simulink model "Beautiful_powertrain"  (R2024a)
settings: Solver=ode3  StartTime=0.0  StopTime=40  FixedStep=0.001  RelTol=1e-3
model workspace (MAT data in the model file):
  C_Aero_drag = 0.28
  C_rolling_resistance = 0.01
  C_rolling_resitance = 0.01
  C_viscous_damping = 0.02
  Damping_coef = 50
  Gear_ratio = 10
  J_vehicle = 2.56328
  Motor_no_load_speed = 16000
  Motor_rated_load = 150000
  Motor_rated_speed = 9000
  Motor_rotor_damping = 0.02
  Motor_rotor_inertia = 0.05
  Motor_voltage = 450
  Slope = 0
  Vehicle_Wheel_Radius = 0.358
  Vehicle_frontal_area = 2.56
  Vehicle_mass = 2000
values from neighbouring files (symbols this model uses):
  s = sprintf('    [N_diangostic_2.m]
undefined symbols (not defined in the file or in its folder): battery_builder_rtmsupport, gcbh
libraries: Batteries_lib x36, fl_lib x31, nesl_utility x24, ee_lib x3, autolibshared x2, rllib x2, sdl_lib x1
(part 2 of 6)

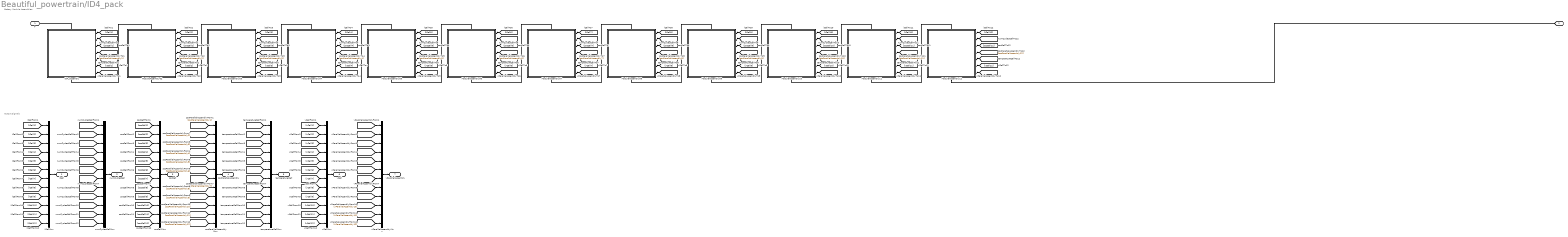
== system Beautiful_powertrain/ID4_pack ==
  note: Output Signals
  note: Battery Module Assemblies
  ID4_Assembly : Subsystem  LoadFcn=battery_builder_rtmsupport('loadfcn',gcbh);
      settings: CopyFcn=battery_builder_rtmsupport('copyfcn',gcbh);  PreCopyFcn=battery_builder_rtmsupport('precopyfcn',gcbh);  PreDeleteFcn=battery_builder_rtmsupport('predeletefcn',gcbh);  PortSchema="{\"entries\":[{\"content\":{\"sides\":[{\"content\":{\"connectorIds\":[\"LConn1\"]},\"type\":\"ConnectorPlacement.EquallySpacedRectSide\",\"uuid\":\"ff832d46-24c2-48f3-9ca2-acbc79ffea0e\"},{\"content\":{\"connectorIds\":[\"RConn1\"],\"side\":\"RIGHT\"},\"type\":\"ConnectorPlacement.EquallySpacedRectSide\",\"uuid\":\"f1f3b13c-36d9-4e7c-bb66-ad6aba201785\"},{\"content\":{\"side\":\"TOP\"},\"type\":\"ConnectorPlacement.EquallySpacedRectSide\",\"uuid\":\"497ed55c-0d21-4aaa-b04e-04d199c99403\"},{\"content\":{\"connectorIds\":[\"Out1\",\"Out2\",\"Out3\",\"Out4\",\"Out5\",\"Out6\",\"Out7\"],\"side\":\"BOTTOM\"},\"type\":\"ConnectorPlacement.EquallySpacedRectSide\",\"uuid\":\"076cd1de-5daa-42e2-9426-d52e4d178271\"}]},\"type\":\"ConnectorPlacement.EquallySpacedConnector\",\"uuid\":\"b44e404e-c709-4efd-83da-0fbfd4cccfd0\"}],\"packageUris\":[\"http://schema.mathworks.com/mf0/Connector/R2020b\"],\"version\":\"1.0\"}"
      mask Display: image('$imagefile')
  ModuleAssembly02 : Subsystem  LoadFcn=battery_builder_rtmsupport('loadfcn',gcbh);
      settings: CopyFcn=battery_builder_rtmsupport('copyfcn',gcbh);  PreCopyFcn=battery_builder_rtmsupport('precopyfcn',gcbh);  PreDeleteFcn=battery_builder_rtmsupport('predeletefcn',gcbh);  PortSchema="{\"entries\":[{\"content\":{\"sides\":[{\"content\":{\"connectorIds\":[\"LConn1\"]},\"type\":\"ConnectorPlacement.EquallySpacedRectSide\",\"uuid\":\"ff832d46-24c2-48f3-9ca2-acbc79ffea0e\"},{\"content\":{\"connectorIds\":[\"RConn1\"],\"side\":\"RIGHT\"},\"type\":\"ConnectorPlacement.EquallySpacedRectSide\",\"uuid\":\"f1f3b13c-36d9-4e7c-bb66-ad6aba201785\"},{\"content\":{\"side\":\"TOP\"},\"type\":\"ConnectorPlacement.EquallySpacedRectSide\",\"uuid\":\"497ed55c-0d21-4aaa-b04e-04d199c99403\"},{\"content\":{\"connectorIds\":[\"Out1\",\"Out2\",\"Out3\",\"Out4\",\"Out5\",\"Out6\",\"Out7\"],\"side\":\"BOTTOM\"},\"type\":\"ConnectorPlacement.EquallySpacedRectSide\",\"uuid\":\"076cd1de-5daa-42e2-9426-d52e4d178271\"}]},\"type\":\"ConnectorPlacement.EquallySpacedConnector\",\"uuid\":\"b44e404e-c709-4efd-83da-0fbfd4cccfd0\"}],\"packageUris\":[\"http://schema.mathworks.com/mf0/Connector/R2020b\"],\"version\":\"1.0\"}"
      mask Display: image('$imagefile')
  ModuleAssembly03 : Subsystem  LoadFcn=battery_builder_rtmsupport('loadfcn',gcbh);
      settings: CopyFcn=battery_builder_rtmsupport('copyfcn',gcbh);  PreCopyFcn=battery_builder_rtmsupport('precopyfcn',gcbh);  PreDeleteFcn=battery_builder_rtmsupport('predeletefcn',gcbh);  PortSchema="{\"entries\":[{\"content\":{\"sides\":[{\"content\":{\"connectorIds\":[\"LConn1\"]},\"type\":\"ConnectorPlacement.EquallySpacedRectSide\",\"uuid\":\"ff832d46-24c2-48f3-9ca2-acbc79ffea0e\"},{\"content\":{\"connectorIds\":[\"RConn1\"],\"side\":\"RIGHT\"},\"type\":\"ConnectorPlacement.EquallySpacedRectSide\",\"uuid\":\"f1f3b13c-36d9-4e7c-bb66-ad6aba201785\"},{\"content\":{\"side\":\"TOP\"},\"type\":\"ConnectorPlacement.EquallySpacedRectSide\",\"uuid\":\"497ed55c-0d21-4aaa-b04e-04d199c99403\"},{\"content\":{\"connectorIds\":[\"Out1\",\"Out2\",\"Out3\",\"Out4\",\"Out5\",\"Out6\",\"Out7\"],\"side\":\"BOTTOM\"},\"type\":\"ConnectorPlacement.EquallySpacedRectSide\",\"uuid\":\"076cd1de-5daa-42e2-9426-d52e4d178271\"}]},\"type\":\"ConnectorPlacement.EquallySpacedConnector\",\"uuid\":\"b44e404e-c709-4efd-83da-0fbfd4cccfd0\"}],\"packageUris\":[\"http://schema.mathworks.com/mf0/Connector/R2020b\"],\"version\":\"1.0\"}"
      mask Display: image('$imagefile')
  ModuleAssembly04 : Subsystem  LoadFcn=battery_builder_rtmsupport('loadfcn',gcbh);
      settings: CopyFcn=battery_builder_rtmsupport('copyfcn',gcbh);  PreCopyFcn=battery_builder_rtmsupport('precopyfcn',gcbh);  PreDeleteFcn=battery_builder_rtmsupport('predeletefcn',gcbh);  PortSchema="{\"entries\":[{\"content\":{\"sides\":[{\"content\":{\"connectorIds\":[\"LConn1\"]},\"type\":\"ConnectorPlacement.EquallySpacedRectSide\",\"uuid\":\"ff832d46-24c2-48f3-9ca2-acbc79ffea0e\"},{\"content\":{\"connectorIds\":[\"RConn1\"],\"side\":\"RIGHT\"},\"type\":\"ConnectorPlacement.EquallySpacedRectSide\",\"uuid\":\"f1f3b13c-36d9-4e7c-bb66-ad6aba201785\"},{\"content\":{\"side\":\"TOP\"},\"type\":\"ConnectorPlacement.EquallySpacedRectSide\",\"uuid\":\"497ed55c-0d21-4aaa-b04e-04d199c99403\"},{\"content\":{\"connectorIds\":[\"Out1\",\"Out2\",\"Out3\",\"Out4\",\"Out5\",\"Out6\",\"Out7\"],\"side\":\"BOTTOM\"},\"type\":\"ConnectorPlacement.EquallySpacedRectSide\",\"uuid\":\"076cd1de-5daa-42e2-9426-d52e4d178271\"}]},\"type\":\"ConnectorPlacement.EquallySpacedConnector\",\"uuid\":\"b44e404e-c709-4efd-83da-0fbfd4cccfd0\"}],\"packageUris\":[\"http://schema.mathworks.com/mf0/Connector/R2020b\"],\"version\":\"1.0\"}"
      mask Display: image('$imagefile')
  ModuleAssembly05 : Subsystem  LoadFcn=battery_builder_rtmsupport('loadfcn',gcbh);
      settings: CopyFcn=battery_builder_rtmsupport('copyfcn',gcbh);  PreCopyFcn=battery_builder_rtmsupport('precopyfcn',gcbh);  PreDeleteFcn=battery_builder_rtmsupport('predeletefcn',gcbh);  PortSchema="{\"entries\":[{\"content\":{\"sides\":[{\"content\":{\"connectorIds\":[\"LConn1\"]},\"type\":\"ConnectorPlacement.EquallySpacedRectSide\",\"uuid\":\"ff832d46-24c2-48f3-9ca2-acbc79ffea0e\"},{\"content\":{\"connectorIds\":[\"RConn1\"],\"side\":\"RIGHT\"},\"type\":\"ConnectorPlacement.EquallySpacedRectSide\",\"uuid\":\"f1f3b13c-36d9-4e7c-bb66-ad6aba201785\"},{\"content\":{\"side\":\"TOP\"},\"type\":\"ConnectorPlacement.EquallySpacedRectSide\",\"uuid\":\"497ed55c-0d21-4aaa-b04e-04d199c99403\"},{\"content\":{\"connectorIds\":[\"Out1\",\"Out2\",\"Out3\",\"Out4\",\"Out5\",\"Out6\",\"Out7\"],\"side\":\"BOTTOM\"},\"type\":\"ConnectorPlacement.EquallySpacedRectSide\",\"uuid\":\"076cd1de-5daa-42e2-9426-d52e4d178271\"}]},\"type\":\"ConnectorPlacement.EquallySpacedConnector\",\"uuid\":\"b44e404e-c709-4efd-83da-0fbfd4cccfd0\"}],\"packageUris\":[\"http://schema.mathworks.com/mf0/Connector/R2020b\"],\"version\":\"1.0\"}"
      mask Display: image('$imagefile')
  ModuleAssembly06 : Subsystem  LoadFcn=battery_builder_rtmsupport('loadfcn',gcbh);
      settings: CopyFcn=battery_builder_rtmsupport('copyfcn',gcbh);  PreCopyFcn=battery_builder_rtmsupport('precopyfcn',gcbh);  PreDeleteFcn=battery_builder_rtmsupport('predeletefcn',gcbh);  PortSchema="{\"entries\":[{\"content\":{\"sides\":[{\"content\":{\"connectorIds\":[\"LConn1\"]},\"type\":\"ConnectorPlacement.EquallySpacedRectSide\",\"uuid\":\"ff832d46-24c2-48f3-9ca2-acbc79ffea0e\"},{\"content\":{\"connectorIds\":[\"RConn1\"],\"side\":\"RIGHT\"},\"type\":\"ConnectorPlacement.EquallySpacedRectSide\",\"uuid\":\"f1f3b13c-36d9-4e7c-bb66-ad6aba201785\"},{\"content\":{\"side\":\"TOP\"},\"type\":\"ConnectorPlacement.EquallySpacedRectSide\",\"uuid\":\"497ed55c-0d21-4aaa-b04e-04d199c99403\"},{\"content\":{\"connectorIds\":[\"Out1\",\"Out2\",\"Out3\",\"Out4\",\"Out5\",\"Out6\",\"Out7\"],\"side\":\"BOTTOM\"},\"type\":\"ConnectorPlacement.EquallySpacedRectSide\",\"uuid\":\"076cd1de-5daa-42e2-9426-d52e4d178271\"}]},\"type\":\"ConnectorPlacement.EquallySpacedConnector\",\"uuid\":\"b44e404e-c709-4efd-83da-0fbfd4cccfd0\"}],\"packageUris\":[\"http://schema.mathworks.com/mf0/Connector/R2020b\"],\"version\":\"1.0\"}"
      mask Display: image('$imagefile')
  ModuleAssembly07 : Subsystem  LoadFcn=battery_builder_rtmsupport('loadfcn',gcbh);
      settings: CopyFcn=battery_builder_rtmsupport('copyfcn',gcbh);  PreCopyFcn=battery_builder_rtmsupport('precopyfcn',gcbh);  PreDeleteFcn=battery_builder_rtmsupport('predeletefcn',gcbh);  PortSchema="{\"entries\":[{\"content\":{\"sides\":[{\"content\":{\"connectorIds\":[\"LConn1\"]},\"type\":\"ConnectorPlacement.EquallySpacedRectSide\",\"uuid\":\"ff832d46-24c2-48f3-9ca2-acbc79ffea0e\"},{\"content\":{\"connectorIds\":[\"RConn1\"],\"side\":\"RIGHT\"},\"type\":\"ConnectorPlacement.EquallySpacedRectSide\",\"uuid\":\"f1f3b13c-36d9-4e7c-bb66-ad6aba201785\"},{\"content\":{\"side\":\"TOP\"},\"type\":\"ConnectorPlacement.EquallySpacedRectSide\",\"uuid\":\"497ed55c-0d21-4aaa-b04e-04d199c99403\"},{\"content\":{\"connectorIds\":[\"Out1\",\"Out2\",\"Out3\",\"Out4\",\"Out5\",\"Out6\",\"Out7\"],\"side\":\"BOTTOM\"},\"type\":\"ConnectorPlacement.EquallySpacedRectSide\",\"uuid\":\"076cd1de-5daa-42e2-9426-d52e4d178271\"}]},\"type\":\"ConnectorPlacement.EquallySpacedConnector\",\"uuid\":\"b44e404e-c709-4efd-83da-0fbfd4cccfd0\"}],\"packageUris\":[\"http://schema.mathworks.com/mf0/Connector/R2020b\"],\"version\":\"1.0\"}"
      mask Display: image('$imagefile')
  ModuleAssembly08 : Subsystem  LoadFcn=battery_builder_rtmsupport('loadfcn',gcbh);
      settings: CopyFcn=battery_builder_rtmsupport('copyfcn',gcbh);  PreCopyFcn=battery_builder_rtmsupport('precopyfcn',gcbh);  PreDeleteFcn=battery_builder_rtmsupport('predeletefcn',gcbh);  PortSchema="{\"entries\":[{\"content\":{\"sides\":[{\"content\":{\"connectorIds\":[\"LConn1\"]},\"type\":\"ConnectorPlacement.EquallySpacedRectSide\",\"uuid\":\"ff832d46-24c2-48f3-9ca2-acbc79ffea0e\"},{\"content\":{\"connectorIds\":[\"RConn1\"],\"side\":\"RIGHT\"},\"type\":\"ConnectorPlacement.EquallySpacedRectSide\",\"uuid\":\"f1f3b13c-36d9-4e7c-bb66-ad6aba201785\"},{\"content\":{\"side\":\"TOP\"},\"type\":\"ConnectorPlacement.EquallySpacedRectSide\",\"uuid\":\"497ed55c-0d21-4aaa-b04e-04d199c99403\"},{\"content\":{\"connectorIds\":[\"Out1\",\"Out2\",\"Out3\",\"Out4\",\"Out5\",\"Out6\",\"Out7\"],\"side\":\"BOTTOM\"},\"type\":\"ConnectorPlacement.EquallySpacedRectSide\",\"uuid\":\"076cd1de-5daa-42e2-9426-d52e4d178271\"}]},\"type\":\"ConnectorPlacement.EquallySpacedConnector\",\"uuid\":\"b44e404e-c709-4efd-83da-0fbfd4cccfd0\"}],\"packageUris\":[\"http://schema.mathworks.com/mf0/Connector/R2020b\"],\"version\":\"1.0\"}"
      mask Display: image('$imagefile')
  ModuleAssembly09 : Subsystem  LoadFcn=battery_builder_rtmsupport('loadfcn',gcbh);
      settings: CopyFcn=battery_builder_rtmsupport('copyfcn',gcbh);  PreCopyFcn=battery_builder_rtmsupport('precopyfcn',gcbh);  PreDeleteFcn=battery_builder_rtmsupport('predeletefcn',gcbh);  PortSchema="{\"entries\":[{\"content\":{\"sides\":[{\"content\":{\"connectorIds\":[\"LConn1\"]},\"type\":\"ConnectorPlacement.EquallySpacedRectSide\",\"uuid\":\"ff832d46-24c2-48f3-9ca2-acbc79ffea0e\"},{\"content\":{\"connectorIds\":[\"RConn1\"],\"side\":\"RIGHT\"},\"type\":\"ConnectorPlacement.EquallySpacedRectSide\",\"uuid\":\"f1f3b13c-36d9-4e7c-bb66-ad6aba201785\"},{\"content\":{\"side\":\"TOP\"},\"type\":\"ConnectorPlacement.EquallySpacedRectSide\",\"uuid\":\"497ed55c-0d21-4aaa-b04e-04d199c99403\"},{\"content\":{\"connectorIds\":[\"Out1\",\"Out2\",\"Out3\",\"Out4\",\"Out5\",\"Out6\",\"Out7\"],\"side\":\"BOTTOM\"},\"type\":\"ConnectorPlacement.EquallySpacedRectSide\",\"uuid\":\"076cd1de-5daa-42e2-9426-d52e4d178271\"}]},\"type\":\"ConnectorPlacement.EquallySpacedConnector\",\"uuid\":\"b44e404e-c709-4efd-83da-0fbfd4cccfd0\"}],\"packageUris\":[\"http://schema.mathworks.com/mf0/Connector/R2020b\"],\"version\":\"1.0\"}"
      mask Display: image('$imagefile')
  ModuleAssembly10 : Subsystem  LoadFcn=battery_builder_rtmsupport('loadfcn',gcbh);
      settings: CopyFcn=battery_builder_rtmsupport('copyfcn',gcbh);  PreCopyFcn=battery_builder_rtmsupport('precopyfcn',gcbh);  PreDeleteFcn=battery_builder_rtmsupport('predeletefcn',gcbh);  PortSchema="{\"entries\":[{\"content\":{\"sides\":[{\"content\":{\"connectorIds\":[\"LConn1\"]},\"type\":\"ConnectorPlacement.EquallySpacedRectSide\",\"uuid\":\"ff832d46-24c2-48f3-9ca2-acbc79ffea0e\"},{\"content\":{\"connectorIds\":[\"RConn1\"],\"side\":\"RIGHT\"},\"type\":\"ConnectorPlacement.EquallySpacedRectSide\",\"uuid\":\"f1f3b13c-36d9-4e7c-bb66-ad6aba201785\"},{\"content\":{\"side\":\"TOP\"},\"type\":\"ConnectorPlacement.EquallySpacedRectSide\",\"uuid\":\"497ed55c-0d21-4aaa-b04e-04d199c99403\"},{\"content\":{\"connectorIds\":[\"Out1\",\"Out2\",\"Out3\",\"Out4\",\"Out5\",\"Out6\",\"Out7\"],\"side\":\"BOTTOM\"},\"type\":\"ConnectorPlacement.EquallySpacedRectSide\",\"uuid\":\"076cd1de-5daa-42e2-9426-d52e4d178271\"}]},\"type\":\"ConnectorPlacement.EquallySpacedConnector\",\"uuid\":\"b44e404e-c709-4efd-83da-0fbfd4cccfd0\"}],\"packageUris\":[\"http://schema.mathworks.com/mf0/Connector/R2020b\"],\"version\":\"1.0\"}"
      mask Display: image('$imagefile')
  ModuleAssembly11 : Subsystem  LoadFcn=battery_builder_rtmsupport('loadfcn',gcbh);
      settings: CopyFcn=battery_builder_rtmsupport('copyfcn',gcbh);  PreCopyFcn=battery_builder_rtmsupport('precopyfcn',gcbh);  PreDeleteFcn=battery_builder_rtmsupport('predeletefcn',gcbh);  PortSchema="{\"entries\":[{\"content\":{\"sides\":[{\"content\":{\"connectorIds\":[\"LConn1\"]},\"type\":\"ConnectorPlacement.EquallySpacedRectSide\",\"uuid\":\"ff832d46-24c2-48f3-9ca2-acbc79ffea0e\"},{\"content\":{\"connectorIds\":[\"RConn1\"],\"side\":\"RIGHT\"},\"type\":\"ConnectorPlacement.EquallySpacedRectSide\",\"uuid\":\"f1f3b13c-36d9-4e7c-bb66-ad6aba201785\"},{\"content\":{\"side\":\"TOP\"},\"type\":\"ConnectorPlacement.EquallySpacedRectSide\",\"uuid\":\"497ed55c-0d21-4aaa-b04e-04d199c99403\"},{\"content\":{\"connectorIds\":[\"Out1\",\"Out2\",\"Out3\",\"Out4\",\"Out5\",\"Out6\",\"Out7\"],\"side\":\"BOTTOM\"},\"type\":\"ConnectorPlacement.EquallySpacedRectSide\",\"uuid\":\"076cd1de-5daa-42e2-9426-d52e4d178271\"}]},\"type\":\"ConnectorPlacement.EquallySpacedConnector\",\"uuid\":\"b44e404e-c709-4efd-83da-0fbfd4cccfd0\"}],\"packageUris\":[\"http://schema.mathworks.com/mf0/Connector/R2020b\"],\"version\":\"1.0\"}"
      mask Display: image('$imagefile')
  ModuleAssembly12 : Subsystem  LoadFcn=battery_builder_rtmsupport('loadfcn',gcbh);
      settings: CopyFcn=battery_builder_rtmsupport('copyfcn',gcbh);  PreCopyFcn=battery_builder_rtmsupport('precopyfcn',gcbh);  PreDeleteFcn=battery_builder_rtmsupport('predeletefcn',gcbh);  PortSchema="{\"entries\":[{\"content\":{\"sides\":[{\"content\":{\"connectorIds\":[\"LConn1\"]},\"type\":\"ConnectorPlacement.EquallySpacedRectSide\",\"uuid\":\"ff832d46-24c2-48f3-9ca2-acbc79ffea0e\"},{\"content\":{\"connectorIds\":[\"RConn1\"],\"side\":\"RIGHT\"},\"type\":\"ConnectorPlacement.EquallySpacedRectSide\",\"uuid\":\"f1f3b13c-36d9-4e7c-bb66-ad6aba201785\"},{\"content\":{\"side\":\"TOP\"},\"type\":\"ConnectorPlacement.EquallySpacedRectSide\",\"uuid\":\"497ed55c-0d21-4aaa-b04e-04d199c99403\"},{\"content\":{\"connectorIds\":[\"Out1\",\"Out2\",\"Out3\",\"Out4\",\"Out5\",\"Out6\",\"Out7\"],\"side\":\"BOTTOM\"},\"type\":\"ConnectorPlacement.EquallySpacedRectSide\",\"uuid\":\"076cd1de-5daa-42e2-9426-d52e4d178271\"}]},\"type\":\"ConnectorPlacement.EquallySpacedConnector\",\"uuid\":\"b44e404e-c709-4efd-83da-0fbfd4cccfd0\"}],\"packageUris\":[\"http://schema.mathworks.com/mf0/Connector/R2020b\"],\"version\":\"1.0\"}"
      mask Display: image('$imagefile')
  iCellMux : Mux  Inputs=12
  numCyclesCellMux : Mux  Inputs=12
  socCellMux : Mux  Inputs=12
  socParallelAssemblyMux : Mux  Inputs=12
  temperatureCellMux : Mux  Inputs=12
  vCellMux : Mux  Inputs=12
  vParallelAssemblyMux : Mux  Inputs=12
  + : PMIOPort  Side=Left
  - : PMIOPort  Port=2  Side=Right
  iCell : Outport
  numCyclesCell : Outport  Port=2
  socCell : Outport  Port=3
  socParallelAssembly : Outport  Port=4
  temperatureCell : Outport  Port=5
  vCell : Outport  Port=6
  vParallelAssembly : Outport  Port=7
  wires:
  [vParallelAssembly12] -> vParallelAssemblyMux/12
  ModuleAssembly12/7(vParallelAssembly) -> [vParallelAssembly12]
  [vCell12] -> vCellMux/12
  ModuleAssembly12/6(vCell) -> [vCell12]
  [temperatureCell12] -> temperatureCellMux/12
  ModuleAssembly12/5(temperatureCell) -> [temperatureCell12]
  [socParallelAssembly12] -> socParallelAssemblyMux/12
  ModuleAssembly12/4(socParallelAssembly) -> [socParallelAssembly12]
  [socCell12] -> socCellMux/12
  ModuleAssembly12/3(socCell) -> [socCell12]
  [numCyclesCell12] -> numCyclesCellMux/12
  ModuleAssembly12/2(numCyclesCell) -> [numCyclesCell12]
  [iCell12] -> iCellMux/12
  ModuleAssembly12/1(iCell) -> [iCell12]
  [vParallelAssembly11] -> vParallelAssemblyMux/11
  ModuleAssembly11/7(vParallelAssembly) -> [vParallelAssembly11]
  [vCell11] -> vCellMux/11
  ModuleAssembly11/6(vCell) -> [vCell11]
  [temperatureCell11] -> temperatureCellMux/11
  ModuleAssembly11/5(temperatureCell) -> [temperatureCell11]
  [socParallelAssembly11] -> socParallelAssemblyMux/11
  ModuleAssembly11/4(socParallelAssembly) -> [socParallelAssembly11]
  [socCell11] -> socCellMux/11
  ModuleAssembly11/3(socCell) -> [socCell11]
  [numCyclesCell11] -> numCyclesCellMux/11
  ModuleAssembly11/2(numCyclesCell) -> [numCyclesCell11]
  [iCell11] -> iCellMux/11
  ModuleAssembly11/1(iCell) -> [iCell11]
  [vParallelAssembly10] -> vParallelAssemblyMux/10
  ModuleAssembly10/7(vParallelAssembly) -> [vParallelAssembly10]
  [vCell10] -> vCellMux/10
  ModuleAssembly10/6(vCell) -> [vCell10]
  [temperatureCell10] -> temperatureCellMux/10
  ModuleAssembly10/5(temperatureCell) -> [temperatureCell10]
  [socParallelAssembly10] -> socParallelAssemblyMux/10
  ModuleAssembly10/4(socParallelAssembly) -> [socParallelAssembly10]
  [socCell10] -> socCellMux/10
  ModuleAssembly10/3(socCell) -> [socCell10]
  [numCyclesCell10] -> numCyclesCellMux/10
  ModuleAssembly10/2(numCyclesCell) -> [numCyclesCell10]
  [iCell10] -> iCellMux/10
  ModuleAssembly10/1(iCell) -> [iCell10]
  [vParallelAssembly9] -> vParallelAssemblyMux/9
  ModuleAssembly09/7(vParallelAssembly) -> [vParallelAssembly9]
  [vCell9] -> vCellMux/9
  ModuleAssembly09/6(vCell) -> [vCell9]
  [temperatureCell9] -> temperatureCellMux/9
  ModuleAssembly09/5(temperatureCell) -> [temperatureCell9]
  [socParallelAssembly9] -> socParallelAssemblyMux/9
  ModuleAssembly09/4(socParallelAssembly) -> [socParallelAssembly9]
  [socCell9] -> socCellMux/9
  ModuleAssembly09/3(socCell) -> [socCell9]
  [numCyclesCell9] -> numCyclesCellMux/9
  ModuleAssembly09/2(numCyclesCell) -> [numCyclesCell9]
  [iCell9] -> iCellMux/9
  ModuleAssembly09/1(iCell) -> [iCell9]
  [vParallelAssembly8] -> vParallelAssemblyMux/8
  ModuleAssembly08/7(vParallelAssembly) -> [vParallelAssembly8]
  [vCell8] -> vCellMux/8
  ModuleAssembly08/6(vCell) -> [vCell8]
  [temperatureCell8] -> temperatureCellMux/8
  ModuleAssembly08/5(temperatureCell) -> [temperatureCell8]
  [socParallelAssembly8] -> socParallelAssemblyMux/8
  ModuleAssembly08/4(socParallelAssembly) -> [socParallelAssembly8]
  [socCell8] -> socCellMux/8
  ModuleAssembly08/3(socCell) -> [socCell8]
  [numCyclesCell8] -> numCyclesCellMux/8
  ModuleAssembly08/2(numCyclesCell) -> [numCyclesCell8]
  [iCell8] -> iCellMux/8
  ModuleAssembly08/1(iCell) -> [iCell8]
  [vParallelAssembly7] -> vParallelAssemblyMux/7
  ModuleAssembly07/7(vParallelAssembly) -> [vParallelAssembly7]
  [vCell7] -> vCellMux/7
  ModuleAssembly07/6(vCell) -> [vCell7]
  [temperatureCell7] -> temperatureCellMux/7
  ModuleAssembly07/5(temperatureCell) -> [temperatureCell7]
  [socParallelAssembly7] -> socParallelAssemblyMux/7
  ModuleAssembly07/4(socParallelAssembly) -> [socParallelAssembly7]
  [socCell7] -> socCellMux/7
  ModuleAssembly07/3(socCell) -> [socCell7]
  [numCyclesCell7] -> numCyclesCellMux/7
  ModuleAssembly07/2(numCyclesCell) -> [numCyclesCell7]
  [iCell7] -> iCellMux/7
  ModuleAssembly07/1(iCell) -> [iCell7]
  [vParallelAssembly6] -> vParallelAssemblyMux/6
  ModuleAssembly06/7(vParallelAssembly) -> [vParallelAssembly6]
  [vCell6] -> vCellMux/6
  ModuleAssembly06/6(vCell) -> [vCell6]
  [temperatureCell6] -> temperatureCellMux/6
  ModuleAssembly06/5(temperatureCell) -> [temperatureCell6]
  [socParallelAssembly6] -> socParallelAssemblyMux/6
  ModuleAssembly06/4(socParallelAssembly) -> [socParallelAssembly6]
  [socCell6] -> socCellMux/6
  ModuleAssembly06/3(socCell) -> [socCell6]
  [numCyclesCell6] -> numCyclesCellMux/6
  ModuleAssembly06/2(numCyclesCell) -> [numCyclesCell6]
  [iCell6] -> iCellMux/6
  ModuleAssembly06/1(iCell) -> [iCell6]
  [vParallelAssembly5] -> vParallelAssemblyMux/5
  ModuleAssembly05/7(vParallelAssembly) -> [vParallelAssembly5]
  [vCell5] -> vCellMux/5
  ModuleAssembly05/6(vCell) -> [vCell5]
  [temperatureCell5] -> temperatureCellMux/5
  ModuleAssembly05/5(temperatureCell) -> [temperatureCell5]
  [socParallelAssembly5] -> socParallelAssemblyMux/5
  ModuleAssembly05/4(socParallelAssembly) -> [socParallelAssembly5]
  [socCell5] -> socCellMux/5
  ModuleAssembly05/3(socCell) -> [socCell5]
  [numCyclesCell5] -> numCyclesCellMux/5
  ModuleAssembly05/2(numCyclesCell) -> [numCyclesCell5]
  [iCell5] -> iCellMux/5
  ModuleAssembly05/1(iCell) -> [iCell5]
  [vParallelAssembly4] -> vParallelAssemblyMux/4
  ModuleAssembly04/7(vParallelAssembly) -> [vParallelAssembly4]
  [vCell4] -> vCellMux/4
  ModuleAssembly04/6(vCell) -> [vCell4]
  [temperatureCell4] -> temperatureCellMux/4
  ModuleAssembly04/5(temperatureCell) -> [temperatureCell4]
  [socParallelAssembly4] -> socParallelAssemblyMux/4
  ModuleAssembly04/4(socParallelAssembly) -> [socParallelAssembly4]
  [socCell4] -> socCellMux/4
  ModuleAssembly04/3(socCell) -> [socCell4]
  [numCyclesCell4] -> numCyclesCellMux/4
  ModuleAssembly04/2(numCyclesCell) -> [numCyclesCell4]
  [iCell4] -> iCellMux/4
  ModuleAssembly04/1(iCell) -> [iCell4]
  [vParallelAssembly3] -> vParallelAssemblyMux/3
  ModuleAssembly03/7(vParallelAssembly) -> [vParallelAssembly3]
  [vCell3] -> vCellMux/3
  ModuleAssembly03/6(vCell) -> [vCell3]
  [temperatureCell3] -> temperatureCellMux/3
  ModuleAssembly03/5(temperatureCell) -> [temperatureCell3]
  [socParallelAssembly3] -> socParallelAssemblyMux/3
  ModuleAssembly03/4(socParallelAssembly) -> [socParallelAssembly3]
  [socCell3] -> socCellMux/3
  ModuleAssembly03/3(socCell) -> [socCell3]
  [numCyclesCell3] -> numCyclesCellMux/3
  ModuleAssembly03/2(numCyclesCell) -> [numCyclesCell3]
  [iCell3] -> iCellMux/3
  ModuleAssembly03/1(iCell) -> [iCell3]
  [vParallelAssembly2] -> vParallelAssemblyMux/2
  ModuleAssembly02/7(vParallelAssembly) -> [vParallelAssembly2]
  [vCell2] -> vCellMux/2
  ModuleAssembly02/6(vCell) -> [vCell2]
  [temperatureCell2] -> temperatureCellMux/2
  ModuleAssembly02/5(temperatureCell) -> [temperatureCell2]
  [socParallelAssembly2] -> socParallelAssemblyMux/2
  ModuleAssembly02/4(socParallelAssembly) -> [socParallelAssembly2]
  [socCell2] -> socCellMux/2
  ModuleAssembly02/3(socCell) -> [socCell2]
  [numCyclesCell2] -> numCyclesCellMux/2
  ModuleAssembly02/2(numCyclesCell) -> [numCyclesCell2]
  [iCell2] -> iCellMux/2
  ModuleAssembly02/1(iCell) -> [iCell2]
  [vParallelAssembly1] -> vParallelAssemblyMux/1
  vParallelAssemblyMux/1 -> vParallelAssembly/1
  ID4_Assembly/7(vParallelAssembly) -> [vParallelAssembly1]
  [vCell1] -> vCellMux/1
  vCellMux/1 -> vCell/1
  ID4_Assembly/6(vCell) -> [vCell1]
  [temperatureCell1] -> temperatureCellMux/1
  temperatureCellMux/1 -> temperatureCell/1
  ID4_Assembly/5(temperatureCell) -> [temperatureCell1]
  [socParallelAssembly1] -> socParallelAssemblyMux/1
  socParallelAssemblyMux/1 -> socParallelAssembly/1
  ID4_Assembly/4(socParallelAssembly) -> [socParallelAssembly1]
  [socCell1] -> socCellMux/1
  socCellMux/1 -> socCell/1
  ID4_Assembly/3(socCell) -> [socCell1]
  [numCyclesCell1] -> numCyclesCellMux/1
  numCyclesCellMux/1 -> numCyclesCell/1
  ID4_Assembly/2(numCyclesCell) -> [numCyclesCell1]
  [iCell1] -> iCellMux/1
  iCellMux/1 -> iCell/1
  ID4_Assembly/1(iCell) -> [iCell1]
  connections:
  ModuleAssembly12/RConn1 -- -/RConn1
  ID4_Assembly/LConn1 -- +/RConn1
  ModuleAssembly12/LConn1 -- ModuleAssembly11/RConn1
  ModuleAssembly11/LConn1 -- ModuleAssembly10/RConn1
  ModuleAssembly10/LConn1 -- ModuleAssembly09/RConn1
  ModuleAssembly09/LConn1 -- ModuleAssembly08/RConn1
  ModuleAssembly08/LConn1 -- ModuleAssembly07/RConn1
  ModuleAssembly07/LConn1 -- ModuleAssembly06/RConn1
  ModuleAssembly06/LConn1 -- ModuleAssembly05/RConn1
  ModuleAssembly05/LConn1 -- ModuleAssembly04/RConn1
  ModuleAssembly04/LConn1 -- ModuleAssembly03/RConn1
  ModuleAssembly03/LConn1 -- ModuleAssembly02/RConn1
  ModuleAssembly02/LConn1 -- ID4_Assembly/RConn1

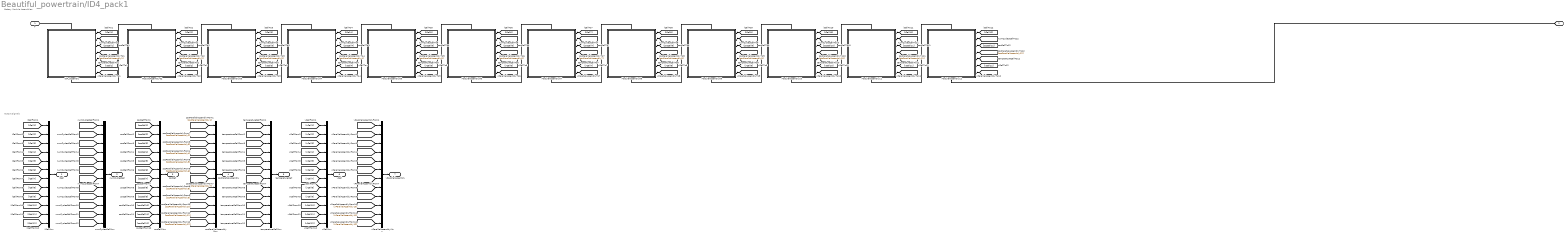
== system Beautiful_powertrain/ID4_pack1 ==
  note: Battery Module Assemblies
  note: Output Signals
  ID4_Assembly : Subsystem  LoadFcn=battery_builder_rtmsupport('loadfcn',gcbh);
      settings: CopyFcn=battery_builder_rtmsupport('copyfcn',gcbh);  PreCopyFcn=battery_builder_rtmsupport('precopyfcn',gcbh);  PreDeleteFcn=battery_builder_rtmsupport('predeletefcn',gcbh);  PortSchema="{\"entries\":[{\"content\":{\"sides\":[{\"content\":{\"connectorIds\":[\"LConn1\"]},\"type\":\"ConnectorPlacement.EquallySpacedRectSide\",\"uuid\":\"ff832d46-24c2-48f3-9ca2-acbc79ffea0e\"},{\"content\":{\"connectorIds\":[\"RConn1\"],\"side\":\"RIGHT\"},\"type\":\"ConnectorPlacement.EquallySpacedRectSide\",\"uuid\":\"f1f3b13c-36d9-4e7c-bb66-ad6aba201785\"},{\"content\":{\"side\":\"TOP\"},\"type\":\"ConnectorPlacement.EquallySpacedRectSide\",\"uuid\":\"497ed55c-0d21-4aaa-b04e-04d199c99403\"},{\"content\":{\"connectorIds\":[\"Out1\",\"Out2\",\"Out3\",\"Out4\",\"Out5\",\"Out6\",\"Out7\"],\"side\":\"BOTTOM\"},\"type\":\"ConnectorPlacement.EquallySpacedRectSide\",\"uuid\":\"076cd1de-5daa-42e2-9426-d52e4d178271\"}]},\"type\":\"ConnectorPlacement.EquallySpacedConnector\",\"uuid\":\"b44e404e-c709-4efd-83da-0fbfd4cccfd0\"}],\"packageUris\":[\"http://schema.mathworks.com/mf0/Connector/R2020b\"],\"version\":\"1.0\"}"
      mask Display: image('$imagefile')
  ModuleAssembly02 : Subsystem  LoadFcn=battery_builder_rtmsupport('loadfcn',gcbh);
      settings: CopyFcn=battery_builder_rtmsupport('copyfcn',gcbh);  PreCopyFcn=battery_builder_rtmsupport('precopyfcn',gcbh);  PreDeleteFcn=battery_builder_rtmsupport('predeletefcn',gcbh);  PortSchema="{\"entries\":[{\"content\":{\"sides\":[{\"content\":{\"connectorIds\":[\"LConn1\"]},\"type\":\"ConnectorPlacement.EquallySpacedRectSide\",\"uuid\":\"ff832d46-24c2-48f3-9ca2-acbc79ffea0e\"},{\"content\":{\"connectorIds\":[\"RConn1\"],\"side\":\"RIGHT\"},\"type\":\"ConnectorPlacement.EquallySpacedRectSide\",\"uuid\":\"f1f3b13c-36d9-4e7c-bb66-ad6aba201785\"},{\"content\":{\"side\":\"TOP\"},\"type\":\"ConnectorPlacement.EquallySpacedRectSide\",\"uuid\":\"497ed55c-0d21-4aaa-b04e-04d199c99403\"},{\"content\":{\"connectorIds\":[\"Out1\",\"Out2\",\"Out3\",\"Out4\",\"Out5\",\"Out6\",\"Out7\"],\"side\":\"BOTTOM\"},\"type\":\"ConnectorPlacement.EquallySpacedRectSide\",\"uuid\":\"076cd1de-5daa-42e2-9426-d52e4d178271\"}]},\"type\":\"ConnectorPlacement.EquallySpacedConnector\",\"uuid\":\"b44e404e-c709-4efd-83da-0fbfd4cccfd0\"}],\"packageUris\":[\"http://schema.mathworks.com/mf0/Connector/R2020b\"],\"version\":\"1.0\"}"
      mask Display: image('$imagefile')
  ModuleAssembly03 : Subsystem  LoadFcn=battery_builder_rtmsupport('loadfcn',gcbh);
      settings: CopyFcn=battery_builder_rtmsupport('copyfcn',gcbh);  PreCopyFcn=battery_builder_rtmsupport('precopyfcn',gcbh);  PreDeleteFcn=battery_builder_rtmsupport('predeletefcn',gcbh);  PortSchema="{\"entries\":[{\"content\":{\"sides\":[{\"content\":{\"connectorIds\":[\"LConn1\"]},\"type\":\"ConnectorPlacement.EquallySpacedRectSide\",\"uuid\":\"ff832d46-24c2-48f3-9ca2-acbc79ffea0e\"},{\"content\":{\"connectorIds\":[\"RConn1\"],\"side\":\"RIGHT\"},\"type\":\"ConnectorPlacement.EquallySpacedRectSide\",\"uuid\":\"f1f3b13c-36d9-4e7c-bb66-ad6aba201785\"},{\"content\":{\"side\":\"TOP\"},\"type\":\"ConnectorPlacement.EquallySpacedRectSide\",\"uuid\":\"497ed55c-0d21-4aaa-b04e-04d199c99403\"},{\"content\":{\"connectorIds\":[\"Out1\",\"Out2\",\"Out3\",\"Out4\",\"Out5\",\"Out6\",\"Out7\"],\"side\":\"BOTTOM\"},\"type\":\"ConnectorPlacement.EquallySpacedRectSide\",\"uuid\":\"076cd1de-5daa-42e2-9426-d52e4d178271\"}]},\"type\":\"ConnectorPlacement.EquallySpacedConnector\",\"uuid\":\"b44e404e-c709-4efd-83da-0fbfd4cccfd0\"}],\"packageUris\":[\"http://schema.mathworks.com/mf0/Connector/R2020b\"],\"version\":\"1.0\"}"
      mask Display: image('$imagefile')
  ModuleAssembly04 : Subsystem  LoadFcn=battery_builder_rtmsupport('loadfcn',gcbh);
      settings: CopyFcn=battery_builder_rtmsupport('copyfcn',gcbh);  PreCopyFcn=battery_builder_rtmsupport('precopyfcn',gcbh);  PreDeleteFcn=battery_builder_rtmsupport('predeletefcn',gcbh);  PortSchema="{\"entries\":[{\"content\":{\"sides\":[{\"content\":{\"connectorIds\":[\"LConn1\"]},\"type\":\"ConnectorPlacement.EquallySpacedRectSide\",\"uuid\":\"ff832d46-24c2-48f3-9ca2-acbc79ffea0e\"},{\"content\":{\"connectorIds\":[\"RConn1\"],\"side\":\"RIGHT\"},\"type\":\"ConnectorPlacement.EquallySpacedRectSide\",\"uuid\":\"f1f3b13c-36d9-4e7c-bb66-ad6aba201785\"},{\"content\":{\"side\":\"TOP\"},\"type\":\"ConnectorPlacement.EquallySpacedRectSide\",\"uuid\":\"497ed55c-0d21-4aaa-b04e-04d199c99403\"},{\"content\":{\"connectorIds\":[\"Out1\",\"Out2\",\"Out3\",\"Out4\",\"Out5\",\"Out6\",\"Out7\"],\"side\":\"BOTTOM\"},\"type\":\"ConnectorPlacement.EquallySpacedRectSide\",\"uuid\":\"076cd1de-5daa-42e2-9426-d52e4d178271\"}]},\"type\":\"ConnectorPlacement.EquallySpacedConnector\",\"uuid\":\"b44e404e-c709-4efd-83da-0fbfd4cccfd0\"}],\"packageUris\":[\"http://schema.mathworks.com/mf0/Connector/R2020b\"],\"version\":\"1.0\"}"
      mask Display: image('$imagefile')
  ModuleAssembly05 : Subsystem  LoadFcn=battery_builder_rtmsupport('loadfcn',gcbh);
      settings: CopyFcn=battery_builder_rtmsupport('copyfcn',gcbh);  PreCopyFcn=battery_builder_rtmsupport('precopyfcn',gcbh);  PreDeleteFcn=battery_builder_rtmsupport('predeletefcn',gcbh);  PortSchema="{\"entries\":[{\"content\":{\"sides\":[{\"content\":{\"connectorIds\":[\"LConn1\"]},\"type\":\"ConnectorPlacement.EquallySpacedRectSide\",\"uuid\":\"ff832d46-24c2-48f3-9ca2-acbc79ffea0e\"},{\"content\":{\"connectorIds\":[\"RConn1\"],\"side\":\"RIGHT\"},\"type\":\"ConnectorPlacement.EquallySpacedRectSide\",\"uuid\":\"f1f3b13c-36d9-4e7c-bb66-ad6aba201785\"},{\"content\":{\"side\":\"TOP\"},\"type\":\"ConnectorPlacement.EquallySpacedRectSide\",\"uuid\":\"497ed55c-0d21-4aaa-b04e-04d199c99403\"},{\"content\":{\"connectorIds\":[\"Out1\",\"Out2\",\"Out3\",\"Out4\",\"Out5\",\"Out6\",\"Out7\"],\"side\":\"BOTTOM\"},\"type\":\"ConnectorPlacement.EquallySpacedRectSide\",\"uuid\":\"076cd1de-5daa-42e2-9426-d52e4d178271\"}]},\"type\":\"ConnectorPlacement.EquallySpacedConnector\",\"uuid\":\"b44e404e-c709-4efd-83da-0fbfd4cccfd0\"}],\"packageUris\":[\"http://schema.mathworks.com/mf0/Connector/R2020b\"],\"version\":\"1.0\"}"
      mask Display: image('$imagefile')
  ModuleAssembly06 : Subsystem  LoadFcn=battery_builder_rtmsupport('loadfcn',gcbh);
      settings: CopyFcn=battery_builder_rtmsupport('copyfcn',gcbh);  PreCopyFcn=battery_builder_rtmsupport('precopyfcn',gcbh);  PreDeleteFcn=battery_builder_rtmsupport('predeletefcn',gcbh);  PortSchema="{\"entries\":[{\"content\":{\"sides\":[{\"content\":{\"connectorIds\":[\"LConn1\"]},\"type\":\"ConnectorPlacement.EquallySpacedRectSide\",\"uuid\":\"ff832d46-24c2-48f3-9ca2-acbc79ffea0e\"},{\"content\":{\"connectorIds\":[\"RConn1\"],\"side\":\"RIGHT\"},\"type\":\"ConnectorPlacement.EquallySpacedRectSide\",\"uuid\":\"f1f3b13c-36d9-4e7c-bb66-ad6aba201785\"},{\"content\":{\"side\":\"TOP\"},\"type\":\"ConnectorPlacement.EquallySpacedRectSide\",\"uuid\":\"497ed55c-0d21-4aaa-b04e-04d199c99403\"},{\"content\":{\"connectorIds\":[\"Out1\",\"Out2\",\"Out3\",\"Out4\",\"Out5\",\"Out6\",\"Out7\"],\"side\":\"BOTTOM\"},\"type\":\"ConnectorPlacement.EquallySpacedRectSide\",\"uuid\":\"076cd1de-5daa-42e2-9426-d52e4d178271\"}]},\"type\":\"ConnectorPlacement.EquallySpacedConnector\",\"uuid\":\"b44e404e-c709-4efd-83da-0fbfd4cccfd0\"}],\"packageUris\":[\"http://schema.mathworks.com/mf0/Connector/R2020b\"],\"version\":\"1.0\"}"
      mask Display: image('$imagefile')
  ModuleAssembly07 : Subsystem  LoadFcn=battery_builder_rtmsupport('loadfcn',gcbh);
      settings: CopyFcn=battery_builder_rtmsupport('copyfcn',gcbh);  PreCopyFcn=battery_builder_rtmsupport('precopyfcn',gcbh);  PreDeleteFcn=battery_builder_rtmsupport('predeletefcn',gcbh);  PortSchema="{\"entries\":[{\"content\":{\"sides\":[{\"content\":{\"connectorIds\":[\"LConn1\"]},\"type\":\"ConnectorPlacement.EquallySpacedRectSide\",\"uuid\":\"ff832d46-24c2-48f3-9ca2-acbc79ffea0e\"},{\"content\":{\"connectorIds\":[\"RConn1\"],\"side\":\"RIGHT\"},\"type\":\"ConnectorPlacement.EquallySpacedRectSide\",\"uuid\":\"f1f3b13c-36d9-4e7c-bb66-ad6aba201785\"},{\"content\":{\"side\":\"TOP\"},\"type\":\"ConnectorPlacement.EquallySpacedRectSide\",\"uuid\":\"497ed55c-0d21-4aaa-b04e-04d199c99403\"},{\"content\":{\"connectorIds\":[\"Out1\",\"Out2\",\"Out3\",\"Out4\",\"Out5\",\"Out6\",\"Out7\"],\"side\":\"BOTTOM\"},\"type\":\"ConnectorPlacement.EquallySpacedRectSide\",\"uuid\":\"076cd1de-5daa-42e2-9426-d52e4d178271\"}]},\"type\":\"ConnectorPlacement.EquallySpacedConnector\",\"uuid\":\"b44e404e-c709-4efd-83da-0fbfd4cccfd0\"}],\"packageUris\":[\"http://schema.mathworks.com/mf0/Connector/R2020b\"],\"version\":\"1.0\"}"
      mask Display: image('$imagefile')
  ModuleAssembly08 : Subsystem  LoadFcn=battery_builder_rtmsupport('loadfcn',gcbh);
      settings: CopyFcn=battery_builder_rtmsupport('copyfcn',gcbh);  PreCopyFcn=battery_builder_rtmsupport('precopyfcn',gcbh);  PreDeleteFcn=battery_builder_rtmsupport('predeletefcn',gcbh);  PortSchema="{\"entries\":[{\"content\":{\"sides\":[{\"content\":{\"connectorIds\":[\"LConn1\"]},\"type\":\"ConnectorPlacement.EquallySpacedRectSide\",\"uuid\":\"ff832d46-24c2-48f3-9ca2-acbc79ffea0e\"},{\"content\":{\"connectorIds\":[\"RConn1\"],\"side\":\"RIGHT\"},\"type\":\"ConnectorPlacement.EquallySpacedRectSide\",\"uuid\":\"f1f3b13c-36d9-4e7c-bb66-ad6aba201785\"},{\"content\":{\"side\":\"TOP\"},\"type\":\"ConnectorPlacement.EquallySpacedRectSide\",\"uuid\":\"497ed55c-0d21-4aaa-b04e-04d199c99403\"},{\"content\":{\"connectorIds\":[\"Out1\",\"Out2\",\"Out3\",\"Out4\",\"Out5\",\"Out6\",\"Out7\"],\"side\":\"BOTTOM\"},\"type\":\"ConnectorPlacement.EquallySpacedRectSide\",\"uuid\":\"076cd1de-5daa-42e2-9426-d52e4d178271\"}]},\"type\":\"ConnectorPlacement.EquallySpacedConnector\",\"uuid\":\"b44e404e-c709-4efd-83da-0fbfd4cccfd0\"}],\"packageUris\":[\"http://schema.mathworks.com/mf0/Connector/R2020b\"],\"version\":\"1.0\"}"
      mask Display: image('$imagefile')
  ModuleAssembly09 : Subsystem  LoadFcn=battery_builder_rtmsupport('loadfcn',gcbh);
      settings: CopyFcn=battery_builder_rtmsupport('copyfcn',gcbh);  PreCopyFcn=battery_builder_rtmsupport('precopyfcn',gcbh);  PreDeleteFcn=battery_builder_rtmsupport('predeletefcn',gcbh);  PortSchema="{\"entries\":[{\"content\":{\"sides\":[{\"content\":{\"connectorIds\":[\"LConn1\"]},\"type\":\"ConnectorPlacement.EquallySpacedRectSide\",\"uuid\":\"ff832d46-24c2-48f3-9ca2-acbc79ffea0e\"},{\"content\":{\"connectorIds\":[\"RConn1\"],\"side\":\"RIGHT\"},\"type\":\"ConnectorPlacement.EquallySpacedRectSide\",\"uuid\":\"f1f3b13c-36d9-4e7c-bb66-ad6aba201785\"},{\"content\":{\"side\":\"TOP\"},\"type\":\"ConnectorPlacement.EquallySpacedRectSide\",\"uuid\":\"497ed55c-0d21-4aaa-b04e-04d199c99403\"},{\"content\":{\"connectorIds\":[\"Out1\",\"Out2\",\"Out3\",\"Out4\",\"Out5\",\"Out6\",\"Out7\"],\"side\":\"BOTTOM\"},\"type\":\"ConnectorPlacement.EquallySpacedRectSide\",\"uuid\":\"076cd1de-5daa-42e2-9426-d52e4d178271\"}]},\"type\":\"ConnectorPlacement.EquallySpacedConnector\",\"uuid\":\"b44e404e-c709-4efd-83da-0fbfd4cccfd0\"}],\"packageUris\":[\"http://schema.mathworks.com/mf0/Connector/R2020b\"],\"version\":\"1.0\"}"
      mask Display: image('$imagefile')
  ModuleAssembly10 : Subsystem  LoadFcn=battery_builder_rtmsupport('loadfcn',gcbh);
      settings: CopyFcn=battery_builder_rtmsupport('copyfcn',gcbh);  PreCopyFcn=battery_builder_rtmsupport('precopyfcn',gcbh);  PreDeleteFcn=battery_builder_rtmsupport('predeletefcn',gcbh);  PortSchema="{\"entries\":[{\"content\":{\"sides\":[{\"content\":{\"connectorIds\":[\"LConn1\"]},\"type\":\"ConnectorPlacement.EquallySpacedRectSide\",\"uuid\":\"ff832d46-24c2-48f3-9ca2-acbc79ffea0e\"},{\"content\":{\"connectorIds\":[\"RConn1\"],\"side\":\"RIGHT\"},\"type\":\"ConnectorPlacement.EquallySpacedRectSide\",\"uuid\":\"f1f3b13c-36d9-4e7c-bb66-ad6aba201785\"},{\"content\":{\"side\":\"TOP\"},\"type\":\"ConnectorPlacement.EquallySpacedRectSide\",\"uuid\":\"497ed55c-0d21-4aaa-b04e-04d199c99403\"},{\"content\":{\"connectorIds\":[\"Out1\",\"Out2\",\"Out3\",\"Out4\",\"Out5\",\"Out6\",\"Out7\"],\"side\":\"BOTTOM\"},\"type\":\"ConnectorPlacement.EquallySpacedRectSide\",\"uuid\":\"076cd1de-5daa-42e2-9426-d52e4d178271\"}]},\"type\":\"ConnectorPlacement.EquallySpacedConnector\",\"uuid\":\"b44e404e-c709-4efd-83da-0fbfd4cccfd0\"}],\"packageUris\":[\"http://schema.mathworks.com/mf0/Connector/R2020b\"],\"version\":\"1.0\"}"
      mask Display: image('$imagefile')
  ModuleAssembly11 : Subsystem  LoadFcn=battery_builder_rtmsupport('loadfcn',gcbh);
      settings: CopyFcn=battery_builder_rtmsupport('copyfcn',gcbh);  PreCopyFcn=battery_builder_rtmsupport('precopyfcn',gcbh);  PreDeleteFcn=battery_builder_rtmsupport('predeletefcn',gcbh);  PortSchema="{\"entries\":[{\"content\":{\"sides\":[{\"content\":{\"connectorIds\":[\"LConn1\"]},\"type\":\"ConnectorPlacement.EquallySpacedRectSide\",\"uuid\":\"ff832d46-24c2-48f3-9ca2-acbc79ffea0e\"},{\"content\":{\"connectorIds\":[\"RConn1\"],\"side\":\"RIGHT\"},\"type\":\"ConnectorPlacement.EquallySpacedRectSide\",\"uuid\":\"f1f3b13c-36d9-4e7c-bb66-ad6aba201785\"},{\"content\":{\"side\":\"TOP\"},\"type\":\"ConnectorPlacement.EquallySpacedRectSide\",\"uuid\":\"497ed55c-0d21-4aaa-b04e-04d199c99403\"},{\"content\":{\"connectorIds\":[\"Out1\",\"Out2\",\"Out3\",\"Out4\",\"Out5\",\"Out6\",\"Out7\"],\"side\":\"BOTTOM\"},\"type\":\"ConnectorPlacement.EquallySpacedRectSide\",\"uuid\":\"076cd1de-5daa-42e2-9426-d52e4d178271\"}]},\"type\":\"ConnectorPlacement.EquallySpacedConnector\",\"uuid\":\"b44e404e-c709-4efd-83da-0fbfd4cccfd0\"}],\"packageUris\":[\"http://schema.mathworks.com/mf0/Connector/R2020b\"],\"version\":\"1.0\"}"
      mask Display: image('$imagefile')
  ModuleAssembly12 : Subsystem  LoadFcn=battery_builder_rtmsupport('loadfcn',gcbh);
      settings: CopyFcn=battery_builder_rtmsupport('copyfcn',gcbh);  PreCopyFcn=battery_builder_rtmsupport('precopyfcn',gcbh);  PreDeleteFcn=battery_builder_rtmsupport('predeletefcn',gcbh);  PortSchema="{\"entries\":[{\"content\":{\"sides\":[{\"content\":{\"connectorIds\":[\"LConn1\"]},\"type\":\"ConnectorPlacement.EquallySpacedRectSide\",\"uuid\":\"ff832d46-24c2-48f3-9ca2-acbc79ffea0e\"},{\"content\":{\"connectorIds\":[\"RConn1\"],\"side\":\"RIGHT\"},\"type\":\"ConnectorPlacement.EquallySpacedRectSide\",\"uuid\":\"f1f3b13c-36d9-4e7c-bb66-ad6aba201785\"},{\"content\":{\"side\":\"TOP\"},\"type\":\"ConnectorPlacement.EquallySpacedRectSide\",\"uuid\":\"497ed55c-0d21-4aaa-b04e-04d199c99403\"},{\"content\":{\"connectorIds\":[\"Out1\",\"Out2\",\"Out3\",\"Out4\",\"Out5\",\"Out6\",\"Out7\"],\"side\":\"BOTTOM\"},\"type\":\"ConnectorPlacement.EquallySpacedRectSide\",\"uuid\":\"076cd1de-5daa-42e2-9426-d52e4d178271\"}]},\"type\":\"ConnectorPlacement.EquallySpacedConnector\",\"uuid\":\"b44e404e-c709-4efd-83da-0fbfd4cccfd0\"}],\"packageUris\":[\"http://schema.mathworks.com/mf0/Connector/R2020b\"],\"version\":\"1.0\"}"
      mask Display: image('$imagefile')
  iCellMux : Mux  Inputs=12
  numCyclesCellMux : Mux  Inputs=12
  socCellMux : Mux  Inputs=12
  socParallelAssemblyMux : Mux  Inputs=12
  temperatureCellMux : Mux  Inputs=12
  vCellMux : Mux  Inputs=12
  vParallelAssemblyMux : Mux  Inputs=12
  + : PMIOPort  Side=Left
  - : PMIOPort  Port=2  Side=Right
  iCell : Outport
  numCyclesCell : Outport  Port=2
  socCell : Outport  Port=3
  socParallelAssembly : Outport  Port=4
  temperatureCell : Outport  Port=5
  vCell : Outport  Port=6
  vParallelAssembly : Outport  Port=7
  wires:
  ID4_Assembly/1(iCell) -> [iCell1]
  iCellMux/1 -> iCell/1
  [iCell1] -> iCellMux/1
  ID4_Assembly/2(numCyclesCell) -> [numCyclesCell1]
  numCyclesCellMux/1 -> numCyclesCell/1
  [numCyclesCell1] -> numCyclesCellMux/1
  ID4_Assembly/3(socCell) -> [socCell1]
  socCellMux/1 -> socCell/1
  [socCell1] -> socCellMux/1
  ID4_Assembly/4(socParallelAssembly) -> [socParallelAssembly1]
  socParallelAssemblyMux/1 -> socParallelAssembly/1
  [socParallelAssembly1] -> socParallelAssemblyMux/1
  ID4_Assembly/5(temperatureCell) -> [temperatureCell1]
  temperatureCellMux/1 -> temperatureCell/1
  [temperatureCell1] -> temperatureCellMux/1
  ID4_Assembly/6(vCell) -> [vCell1]
  vCellMux/1 -> vCell/1
  [vCell1] -> vCellMux/1
  ID4_Assembly/7(vParallelAssembly) -> [vParallelAssembly1]
  vParallelAssemblyMux/1 -> vParallelAssembly/1
  [vParallelAssembly1] -> vParallelAssemblyMux/1
  ModuleAssembly02/1(iCell) -> [iCell2]
  [iCell2] -> iCellMux/2
  ModuleAssembly02/2(numCyclesCell) -> [numCyclesCell2]
  [numCyclesCell2] -> numCyclesCellMux/2
  ModuleAssembly02/3(socCell) -> [socCell2]
  [socCell2] -> socCellMux/2
  ModuleAssembly02/4(socParallelAssembly) -> [socParallelAssembly2]
  [socParallelAssembly2] -> socParallelAssemblyMux/2
  ModuleAssembly02/5(temperatureCell) -> [temperatureCell2]
  [temperatureCell2] -> temperatureCellMux/2
  ModuleAssembly02/6(vCell) -> [vCell2]
  [vCell2] -> vCellMux/2
  ModuleAssembly02/7(vParallelAssembly) -> [vParallelAssembly2]
  [vParallelAssembly2] -> vParallelAssemblyMux/2
  ModuleAssembly03/1(iCell) -> [iCell3]
  [iCell3] -> iCellMux/3
  ModuleAssembly03/2(numCyclesCell) -> [numCyclesCell3]
  [numCyclesCell3] -> numCyclesCellMux/3
  ModuleAssembly03/3(socCell) -> [socCell3]
  [socCell3] -> socCellMux/3
  ModuleAssembly03/4(socParallelAssembly) -> [socParallelAssembly3]
  [socParallelAssembly3] -> socParallelAssemblyMux/3
  ModuleAssembly03/5(temperatureCell) -> [temperatureCell3]
  [temperatureCell3] -> temperatureCellMux/3
  ModuleAssembly03/6(vCell) -> [vCell3]
  [vCell3] -> vCellMux/3
  ModuleAssembly03/7(vParallelAssembly) -> [vParallelAssembly3]
  [vParallelAssembly3] -> vParallelAssemblyMux/3
  ModuleAssembly04/1(iCell) -> [iCell4]
  [iCell4] -> iCellMux/4
  ModuleAssembly04/2(numCyclesCell) -> [numCyclesCell4]
  [numCyclesCell4] -> numCyclesCellMux/4
  ModuleAssembly04/3(socCell) -> [socCell4]
  [socCell4] -> socCellMux/4
  ModuleAssembly04/4(socParallelAssembly) -> [socParallelAssembly4]
  [socParallelAssembly4] -> socParallelAssemblyMux/4
  ModuleAssembly04/5(temperatureCell) -> [temperatureCell4]
  [temperatureCell4] -> temperatureCellMux/4
  ModuleAssembly04/6(vCell) -> [vCell4]
  [vCell4] -> vCellMux/4
  ModuleAssembly04/7(vParallelAssembly) -> [vParallelAssembly4]
  [vParallelAssembly4] -> vParallelAssemblyMux/4
  ModuleAssembly05/1(iCell) -> [iCell5]
  [iCell5] -> iCellMux/5
  ModuleAssembly05/2(numCyclesCell) -> [numCyclesCell5]
  [numCyclesCell5] -> numCyclesCellMux/5
  ModuleAssembly05/3(socCell) -> [socCell5]
  [socCell5] -> socCellMux/5
  ModuleAssembly05/4(socParallelAssembly) -> [socParallelAssembly5]
  [socParallelAssembly5] -> socParallelAssemblyMux/5
  ModuleAssembly05/5(temperatureCell) -> [temperatureCell5]
  [temperatureCell5] -> temperatureCellMux/5
  ModuleAssembly05/6(vCell) -> [vCell5]
  [vCell5] -> vCellMux/5
  ModuleAssembly05/7(vParallelAssembly) -> [vParallelAssembly5]
  [vParallelAssembly5] -> vParallelAssemblyMux/5
  ModuleAssembly06/1(iCell) -> [iCell6]
  [iCell6] -> iCellMux/6
  ModuleAssembly06/2(numCyclesCell) -> [numCyclesCell6]
  [numCyclesCell6] -> numCyclesCellMux/6
  ModuleAssembly06/3(socCell) -> [socCell6]
  [socCell6] -> socCellMux/6
  ModuleAssembly06/4(socParallelAssembly) -> [socParallelAssembly6]
  [socParallelAssembly6] -> socParallelAssemblyMux/6
  ModuleAssembly06/5(temperatureCell) -> [temperatureCell6]
  [temperatureCell6] -> temperatureCellMux/6
  ModuleAssembly06/6(vCell) -> [vCell6]
  [vCell6] -> vCellMux/6
  ModuleAssembly06/7(vParallelAssembly) -> [vParallelAssembly6]
  [vParallelAssembly6] -> vParallelAssemblyMux/6
  ModuleAssembly07/1(iCell) -> [iCell7]
  [iCell7] -> iCellMux/7
  ModuleAssembly07/2(numCyclesCell) -> [numCyclesCell7]
  [numCyclesCell7] -> numCyclesCellMux/7
  ModuleAssembly07/3(socCell) -> [socCell7]
  [socCell7] -> socCellMux/7
  ModuleAssembly07/4(socParallelAssembly) -> [socParallelAssembly7]
  [socParallelAssembly7] -> socParallelAssemblyMux/7
  ModuleAssembly07/5(temperatureCell) -> [temperatureCell7]
  [temperatureCell7] -> temperatureCellMux/7
  ModuleAssembly07/6(vCell) -> [vCell7]
  [vCell7] -> vCellMux/7
  ModuleAssembly07/7(vParallelAssembly) -> [vParallelAssembly7]
  [vParallelAssembly7] -> vParallelAssemblyMux/7
  ModuleAssembly08/1(iCell) -> [iCell8]
  [iCell8] -> iCellMux/8
  ModuleAssembly08/2(numCyclesCell) -> [numCyclesCell8]
  [numCyclesCell8] -> numCyclesCellMux/8
  ModuleAssembly08/3(socCell) -> [socCell8]
  [socCell8] -> socCellMux/8
  ModuleAssembly08/4(socParallelAssembly) -> [socParallelAssembly8]
  [socParallelAssembly8] -> socParallelAssemblyMux/8
  ModuleAssembly08/5(temperatureCell) -> [temperatureCell8]
  [temperatureCell8] -> temperatureCellMux/8
  ModuleAssembly08/6(vCell) -> [vCell8]
  [vCell8] -> vCellMux/8
  ModuleAssembly08/7(vParallelAssembly) -> [vParallelAssembly8]
  [vParallelAssembly8] -> vParallelAssemblyMux/8
  ModuleAssembly09/1(iCell) -> [iCell9]
  [iCell9] -> iCellMux/9
  ModuleAssembly09/2(numCyclesCell) -> [numCyclesCell9]
  [numCyclesCell9] -> numCyclesCellMux/9
  ModuleAssembly09/3(socCell) -> [socCell9]
  [socCell9] -> socCellMux/9
  ModuleAssembly09/4(socParallelAssembly) -> [socParallelAssembly9]
  [socParallelAssembly9] -> socParallelAssemblyMux/9
  ModuleAssembly09/5(temperatureCell) -> [temperatureCell9]
  [temperatureCell9] -> temperatureCellMux/9
  ModuleAssembly09/6(vCell) -> [vCell9]
  [vCell9] -> vCellMux/9
  ModuleAssembly09/7(vParallelAssembly) -> [vParallelAssembly9]
  [vParallelAssembly9] -> vParallelAssemblyMux/9
  ModuleAssembly10/1(iCell) -> [iCell10]
  [iCell10] -> iCellMux/10
  ModuleAssembly10/2(numCyclesCell) -> [numCyclesCell10]
  [numCyclesCell10] -> numCyclesCellMux/10
  ModuleAssembly10/3(socCell) -> [socCell10]
  [socCell10] -> socCellMux/10
  ModuleAssembly10/4(socParallelAssembly) -> [socParallelAssembly10]
  [socParallelAssembly10] -> socParallelAssemblyMux/10
  ModuleAssembly10/5(temperatureCell) -> [temperatureCell10]
  [temperatureCell10] -> temperatureCellMux/10
  ModuleAssembly10/6(vCell) -> [vCell10]
  [vCell10] -> vCellMux/10
  ModuleAssembly10/7(vParallelAssembly) -> [vParallelAssembly10]
  [vParallelAssembly10] -> vParallelAssemblyMux/10
  ModuleAssembly11/1(iCell) -> [iCell11]
  [iCell11] -> iCellMux/11
  ModuleAssembly11/2(numCyclesCell) -> [numCyclesCell11]
  [numCyclesCell11] -> numCyclesCellMux/11
  ModuleAssembly11/3(socCell) -> [socCell11]
  [socCell11] -> socCellMux/11
  ModuleAssembly11/4(socParallelAssembly) -> [socParallelAssembly11]
  [socParallelAssembly11] -> socParallelAssemblyMux/11
  ModuleAssembly11/5(temperatureCell) -> [temperatureCell11]
  [temperatureCell11] -> temperatureCellMux/11
  ModuleAssembly11/6(vCell) -> [vCell11]
  [vCell11] -> vCellMux/11
  ModuleAssembly11/7(vParallelAssembly) -> [vParallelAssembly11]
  [vParallelAssembly11] -> vParallelAssemblyMux/11
  ModuleAssembly12/1(iCell) -> [iCell12]
  [iCell12] -> iCellMux/12
  ModuleAssembly12/2(numCyclesCell) -> [numCyclesCell12]
  [numCyclesCell12] -> numCyclesCellMux/12
  ModuleAssembly12/3(socCell) -> [socCell12]
  [socCell12] -> socCellMux/12
  ModuleAssembly12/4(socParallelAssembly) -> [socParallelAssembly12]
  [socParallelAssembly12] -> socParallelAssemblyMux/12
  ModuleAssembly12/5(temperatureCell) -> [temperatureCell12]
  [temperatureCell12] -> temperatureCellMux/12
  ModuleAssembly12/6(vCell) -> [vCell12]
  [vCell12] -> vCellMux/12
  ModuleAssembly12/7(vParallelAssembly) -> [vParallelAssembly12]
  [vParallelAssembly12] -> vParallelAssemblyMux/12
  connections:
  ModuleAssembly02/LConn1 -- ID4_Assembly/RConn1
  ModuleAssembly03/LConn1 -- ModuleAssembly02/RConn1
  ModuleAssembly04/LConn1 -- ModuleAssembly03/RConn1
  ModuleAssembly05/LConn1 -- ModuleAssembly04/RConn1
  ModuleAssembly06/LConn1 -- ModuleAssembly05/RConn1
  ModuleAssembly07/LConn1 -- ModuleAssembly06/RConn1
  ModuleAssembly08/LConn1 -- ModuleAssembly07/RConn1
  ModuleAssembly09/LConn1 -- ModuleAssembly08/RConn1
  ModuleAssembly10/LConn1 -- ModuleAssembly09/RConn1
  ModuleAssembly11/LConn1 -- ModuleAssembly10/RConn1
  ModuleAssembly12/LConn1 -- ModuleAssembly11/RConn1
  ID4_Assembly/LConn1 -- +/RConn1
  ModuleAssembly12/RConn1 -- -/RConn1
